simulink model "autoDrillingLogic"  (R2018b)
settings: Solver=FixedStepDiscrete  StartTime=0.0  StopTime=10.0  RelTol=1e-3
PreLoadFcn:
  | G = 10;
  | Rdrum = 0.25;
  | Np = 5;
  | m_topdrive = 1000;
  | m_drillstring = 22500;
  | Rpulley = Rdrum;
  | 
  | m = m_topdrive + m_drillstring;
  | 
  | % Top/Bottom Distance
  | xtop = 48*0.3048;
  | xbott = 0;
  | 
  | % Maximum Torque/Power of Drive
  | Tmax = 8000*1.36;
  | Pmax = 1500*746;
  | 
  | % Initial Conditions
  | v0 = 0; %m/s
  | x0 = 0; %m
  | 
  | % Gravity
  | g = 9.8;
undefined symbols (not defined in the file): Tssc
libraries: simulink x1
settings Model: Creator=jlesage  LastModifiedBy=jlesage

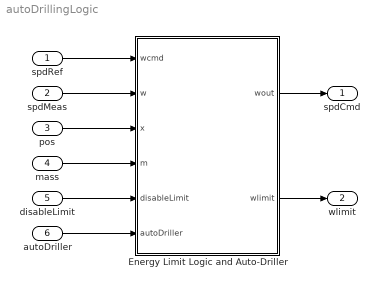
== system autoDrillingLogic ==
  spdRef : Inport  OutMin=-2000  OutMax=2000
  spdMeas : Inport  Port=2  OutMin=-2000  OutMax=2000
  pos : Inport  Port=3  OutMin=-5  OutMax=100
  mass : Inport  Port=4  OutMin=0  OutMax=1e12
  disableLimit : Inport  Port=5  OutDataTypeStr=boolean
  autoDriller : Inport  Port=6  OutDataTypeStr=boolean
  Energy Limit Logic and Auto-Driller : Stateflow chart  TreatAsAtomicUnit=on  SystemSampleTime=Tssc
  spdCmd : Outport
  wlimit : Outport  Port=2
  wires:
  spdRef/1 -> Energy Limit Logic and Auto-Driller/1(wcmd)
  spdMeas/1 -> Energy Limit Logic and Auto-Driller/2(w)
  pos/1 -> Energy Limit Logic and Auto-Driller/3(x)
  mass/1 -> Energy Limit Logic and Auto-Driller/4(m)
  disableLimit/1 -> Energy Limit Logic and Auto-Driller/5(disableLimit)
  autoDriller/1 -> Energy Limit Logic and Auto-Driller/6(autoDriller)
  Energy Limit Logic and Auto-Driller/1(wout) -> spdCmd/1
  Energy Limit Logic and Auto-Driller/2(wlimit) -> wlimit/1

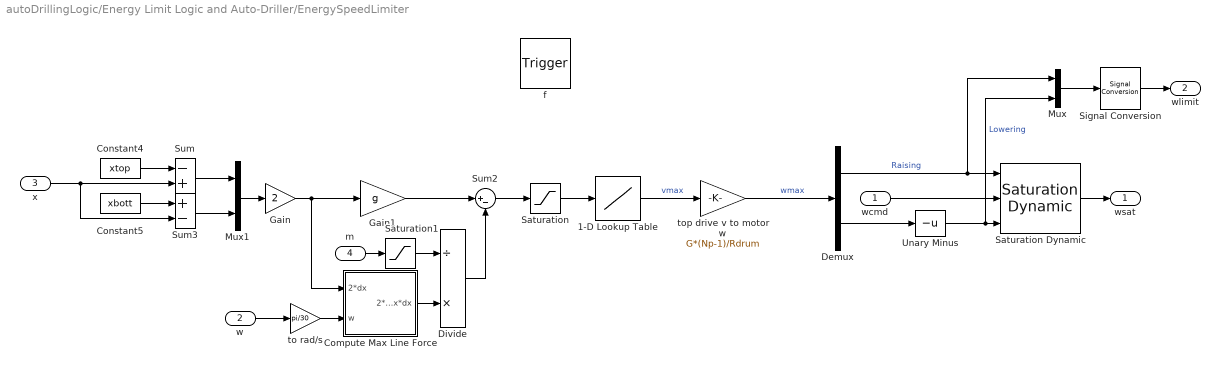
== system autoDrillingLogic/Energy Limit Logic and Auto-Driller/EnergySpeedLimiter ==
  wcmd : Inport  OutDataTypeStr=double  PortDimensions=1
  w : Inport  Port=2  OutDataTypeStr=double  PortDimensions=1
  x : Inport  Port=3  OutDataTypeStr=double  PortDimensions=1
  m : Inport  Port=4  OutDataTypeStr=double  PortDimensions=1
  f : TriggerPort  TriggerType=function-call  VariantControl=(inherit)
      settings: CopyFcn=Stateflow.SLINSF.SimulinkMan.removeBlockPreDeleteFcn  PreDeleteFcn=Stateflow.SLINSF.SimulinkMan.unsafePredeleteFcn
  1-D Lookup Table : Lookup_n-D  NumberOfTableDimensions=1  BreakpointsForDimension1=[0:1000]  Table=sqrt([0:1000])  ExtrapMethod=Clip  InternalRulePriority=Speed  RndMeth=Simplest  InputSameDT=on
  Compute Max Line Force : Subsystem
  Constant4 : Constant  Value=xtop
  Constant5 : Constant  Value=xbott
  Demux : Demux  Outputs=2
  Divide : Product  Inputs=/*
  Gain : Gain  Gain=2
  Gain1 : Gain  Gain=g
  Mux : Mux  Inputs=2
  Mux1 : Mux  Inputs=2
  Saturation : Saturate  UpperLimit=1000  LowerLimit=0
  Saturation Dynamic : simulink/Discontinuities/Saturation Dynamic  OutMin=[]  OutMax=[]  OutDataTypeStr=Inherit: Same as second input  OutDataType=fixdt(1, 16)  OutScaling=2^-10  DoSatur=off
  Saturation1 : Saturate  UpperLimit=1e9  LowerLimit=0.1
  Signal Conversion : SignalConversion  OverrideOpt=off
  Sum : Sum  Inputs=-+
  Sum2 : Sum  Inputs=|+-
  Sum3 : Sum  Inputs=+-
  Unary Minus : UnaryMinus
  to rad/s : Gain  Gain=pi/30
  top drive v to motor w : Gain  Gain=G*(Np-1)/Rdrum
  wsat : Outport
  wlimit : Outport  Port=2
  wires:
  wcmd/1 -> Saturation Dynamic/2
  x/1 -> Sum3/2, Sum/2
  Mux/1 -> Signal Conversion/1
  m/1 -> Saturation1/1
  Constant5/1 -> Sum3/1
  Mux1/1 -> Gain/1
  w/1 -> to rad/s/1
  Sum2/1 -> Saturation/1
  top drive v to motor w/1 -> Demux/1  "wmax"
  Divide/1 -> Sum2/2
  Gain1/1 -> Sum2/1
  Gain/1 -> Compute Max Line Force/1(2*dx), Gain1/1
  Unary Minus/1 -> Mux/2, Saturation Dynamic/3  "Lowering"
  Sum3/1 -> Mux1/2
  Sum/1 -> Mux1/1
  Demux/2 -> Unary Minus/1
  Compute Max Line Force/1(2*Fmax*dx) -> Divide/2
  Saturation/1 -> 1-D Lookup Table/1
  Constant4/1 -> Sum/1
  Demux/1 -> Mux/1, Saturation Dynamic/1  "Raising"
  1-D Lookup Table/1 -> top drive v to motor w/1  "vmax"
  Saturation Dynamic/1 -> wsat/1
  Signal Conversion/1 -> wlimit/1
  to rad/s/1 -> Compute Max Line Force/2(w)
  Saturation1/1 -> Divide/1

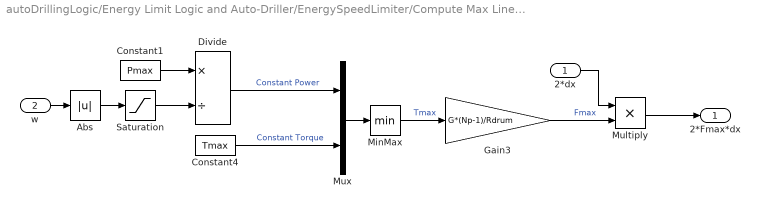
== system autoDrillingLogic/Energy Limit Logic and Auto-Driller/EnergySpeedLimiter/Compute Max Line Force ==
  2*dx : Inport
  w : Inport  Port=2
  Abs : Abs
  Constant1 : Constant  Value=Pmax
  Constant4 : Constant  Value=Tmax
  Divide : Product  Inputs=*/
  Gain3 : Gain  Gain=G*(Np-1)/Rdrum
  MinMax : MinMax
  Multiply : Product
  Mux : Mux  Inputs=2
  Saturation : Saturate  UpperLimit=2000  LowerLimit=0.1
  2*Fmax*dx : Outport
  wires:
  Multiply/1 -> 2*Fmax*dx/1
  2*dx/1 -> Multiply/1
  Gain3/1 -> Multiply/2  "Fmax"
  Constant4/1 -> Mux/2  "Constant Torque"
  Constant1/1 -> Divide/1
  w/1 -> Abs/1
  Saturation/1 -> Divide/2
  Abs/1 -> Saturation/1
  Divide/1 -> Mux/1  "Constant Power"
  Mux/1 -> MinMax/1
  MinMax/1 -> Gain3/1  "Tmax"

== stateflow chart autoDrillingLogic/Energy Limit Logic and Auto-Driller ==
  state Manual
    [wout,wlimit] = EnergySpeedLimiter(wcmd,w,x,m);
  state AutoDriller
    state InitalizeAuto
    state RaiseHoist
      [wout,wlimit] = EnergySpeedLimiter(1000,w,x,m);
    state AddPipeAndMake
      wout = 0;
    state LowerAndDrill
      [wout,wlimit] = EnergySpeedLimiter(-1000,w,x,m);
    state BreakString
      wout = 0;
    (default) -> InitalizeAuto
    InitalizeAuto -> RaiseHoist : [after(2,sec)]
    BreakString -> RaiseHoist : [after(5,sec)]
    RaiseHoist -> AddPipeAndMake : [x >= xtop]
    AddPipeAndMake -> LowerAndDrill : [after(5,sec)]
    LowerAndDrill -> BreakString : [x <= 0.01]
  state DisableLimits
    wout = wcmd;
    wlimit = [2000;-2000];
  state [wsat,wlimit] = EnergySpeedLimiter(wcmd,w,x,m) [function]
  (default) -> Manual
  Manual -> AutoDriller [order 2] : [autoDriller == 1]
  AutoDriller -> Manual : [autoDriller == 0]
  Manual -> DisableLimits [order 1] : [disableLimit == 1]
  DisableLimits -> Manual : [disableLimit == 0]
  data: wcmd function_input double size=1; w function_input double size=1; x function_input double size=1; m function_input double size=1; wsat function_output; wlimit function_output; wcmd input double size=1; w input double size=1; x input double size=1; m input double size=1; disableLimit input boolean size=1; autoDriller input boolean size=1; wout output double size=1; xtop constant double =14.5; wlimit output double size=2
